simulink model "UDPTestSend"  (R2015b)
settings: Solver=VariableStepAuto  StartTime=0.0  StopTime=inf  RelTol=1e-3
libraries: simulink x1, commrandsrc3 x1, dspnetwork x1, aerolibanimutils x1
settings Model: Creator=Ryuu  LastModifiedBy=Ryuu

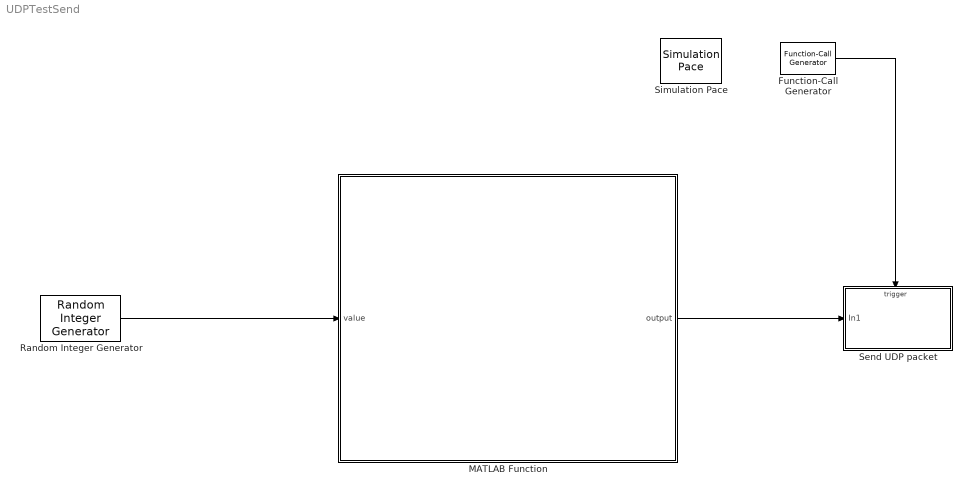
== system UDPTestSend ==
  Function-Call Generator : simulink/Ports & Subsystems/Function-Call Generator  sample_time=.5  numberOfIterations=1
  MATLAB Function : MATLAB Function  TreatAsAtomicUnit=on
  Random Integer Generator : commrandsrc3/Random Integer Generator  SetSize=1000  SeedSource=Auto  Seed=0  SampleTime=0.25  SamplesPerFrame=1  OutputDataType=double  SimulateUsing=Interpreted execution
  Send UDP packet : Subsystem
  Simulation Pace : aerolibanimutils/Simulation Pace  SimulationPace=1  SleepMode=MATLAB Thread  OutputPaceError=off  SampleTime=1/30
  wires:
  Function-Call Generator/1 -> Send UDP packet/Trigger
  Random Integer Generator/1 -> MATLAB Function/1(value)
  MATLAB Function/1(output) -> Send UDP packet/1(In1)

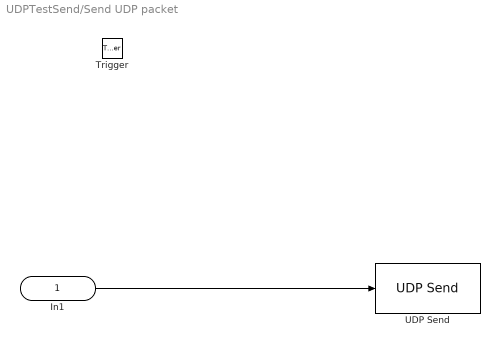
== system UDPTestSend/Send UDP packet ==
  In1 : Inport
  Trigger : TriggerPort  TriggerType=function-call  PortDimensions=1
  UDP Send : dspnetwork/UDP Send  remoteURL='127.0.0.1'  remotePort=25000  localURL='0.0.0.0'  localPortSource=Automatically determine  localPort=-1  sampletime=-1  separateLengthPort=0
  wires:
  In1/1 -> UDP Send/1

== matlab function UDPTestSend/MATLAB Function ==
  data: value input; output output uint8 size=1000
function output = data_serialize(value)
label = 'Test';
type = 'Testsensor';
min = 24;
max = 45;

label_ser = sensor_serialize(label);
type_ser = sensor_serialize(type);
value_ser = sensor_serialize(value);
min_ser = sensor_serialize(min);
max_ser = sensor_serialize(max);


V = length(label_ser);
W = length(type_ser);
X = length(value_ser);
Y = length(min_ser);
Z = length(max_ser);

output = [
    label_ser;
    type_ser;
    value_ser;
    min_ser;
    max_ser;
    ];
end


function m = sensor_serialize(v)
    % dispatch according to type
    if isnumeric(v) 
        m = serialize_numeric(v);
    elseif ischar(v)
        m = serialize_string(v);
    elseif islogical(v)
        m = serialize_logical(v);
	else
		error('Unsupported data type');
    end
end

% single scalar
function m = serialize_scalar(v)
    % Data type & data
    m = [class2tag(class(v)); typecast(v,'uint8').'];
end

% char arrays
function m = serialize_string(v)
    if size(v,1) == 1
        % horizontal string: Type, Length, and Data
        m = [uint8(0); typecast(uint32(length(v)),'uint8').'; uint8(v(:))];
    elseif sum(size(v)) == 0
        % '': special encoding
        m = uint8(200);
    else
        % general char array: Tag & Number of dimensions, Dimensions, Data
        m = [uint8(132); ndims(v); typecast(uint32(size(v)),'uint8').'; uint8(v(:))];
    end
end

% logical arrays
function m = serialize_logical(v)
    % Tag & Number of dimensions, Dimensions, Data
    m = [uint8(133); ndims(v); typecast(uint32(size(v)),'uint8').'; uint8(v(:))];
end

% non-complex and non-sparse numerical matrix
function m = serialize_numeric_simple(v)
    % Tag & Number of dimensions, Dimensions, Data
    m = [16+class2tag(class(v)); ndims(v); typecast(uint32(size(v)),'uint8').'; typecast(v(:).','uint8').'];
end

% Numeric Matrix: can be real/complex, sparse/full, scalar
function m = serialize_numeric(v)
    if issparse(v)
        % Data Type & Dimensions
        m = [uint8(130); typecast(uint64(size(v,1)), 'uint8').'; typecast(uint64(size(v,2)), 'uint8').']; % vectorize
        % Index vectors
        [i,j,s] = find(v);        
        % Real/Complex
        if isreal(v)
            m = [m; serialize_numeric_simple(i); serialize_numeric_simple(j); 1; serialize_numeric_simple(s)];
        else
            m = [m; serialize_numeric_simple(i); serialize_numeric_simple(j); 0; serialize_numeric_simple(real(s)); serialize_numeric_simple(imag(s))];
        end
    elseif ~isreal(v)
        % Data type & contents
        m = [uint8(131); serialize_numeric_simple(real(v)); serialize_numeric_simple(imag(v))];
    elseif isscalar(v)
        % Scalar
        m = serialize_scalar(v);
    else
        % Simple matrix
        m = serialize_numeric_simple(v);
    end
end

% *container* class to byte
function b = class2tag(cls)
	switch cls
		case 'string'
            b = uint8(0);
		case 'double'
			b = uint8(1);
		case 'single'
			b = uint8(2);
		case 'int8'
			b = uint8(3);
		case 'uint8'
			b = uint8(4);
		case 'int16'
			b = uint8(5);
		case 'uint16'
			b = uint8(6);
		case 'int32'
			b = uint8(7);
		case 'uint32'
			b = uint8(8);
		case 'int64'
			b = uint8(9);
		case 'uint64'
			b = uint8(10);
		otherwise
			error('Unknown class');
    end
end
